simulink model "testing_gyro"  (R2016b)
settings: Solver=FixedStepAuto  StartTime=0.0  StopTime=inf  RelTol=1e-3  EnableMultiTasking=on
libraries: legoev3lib x3
settings Model: SimulationMode=external  ExtModeTrigDuration=2  Creator=Shobhit  LastModifiedBy=karanverma
settings SolverCC: PositivePriorityOrder=on
settings OptimizationCC: LifeSpan=1  MaxStackSize=64
settings DebuggingCC: SFUnexpectedBacktrackingDiag=warning  SFNoUnconditionalDefaultTransitionDiag=warning  SFExecutionAtInitializationDiag=none
settings HardwareCC: ProdBitPerPointer=32  ProdBitPerSizeT=32  ProdBitPerPtrDiffT=32  ProdLargestAtomicInteger=Long  ProdWordSize=32  ProdHWDeviceType=ARM Compatible->ARM 9  UseEmbeddedCoderFeatures=off  UseSimulinkCoderFeatures=off
settings RTWCC: SystemTargetFile=ert.tlc  HardwareBoard=LEGO MINDSTORMS EV3  TLCOptions=-aInlineSetEventsForThisBaseRateFcn=TLC_FALSE -aSuppressMultiTaskScheduler=TLC_FALSE -aRateBasedStepFcn=0  TemplateMakefile=ert_default_tmf  Description=Embedded Coder  GenerateReport=on  Toolchain=Sourcery G++ Lite v2009q3  LaunchReport=on
settings CodeAppCC: ForceParamTrailComments=on  OperatorAnnotations=on  MangleLength=10  MATLABSourceComments=on
settings ERTTargetCC: ERTCustomFileBanners=off  SupportContinuousTime=on  SupportNonInlinedSFcns=on  RemoveResetFunc=off  SupportVariableSizeSignals=on  ModelStepFunctionPrototypeControlCompliant=off
settings ConfigComp: CovMetricSettings=dw  CovHtmlReporting=on  CovSaveCumulativeToWorkspaceVar=on  CovSaveSingleToWorkspaceVar=on  CovExternalEMLEnable=off

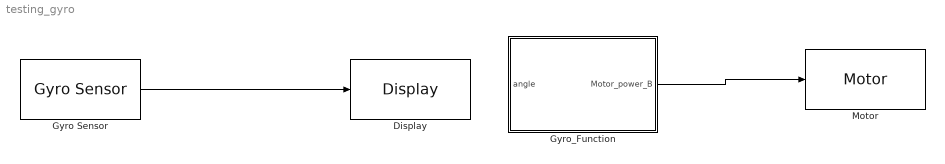
== system testing_gyro ==
  Display : legoev3lib/Display  slcdLine=1  slcdFormat=Decimal
  Gyro Sensor : legoev3lib/Gyro Sensor  portNumber=1  sampleTime=0.1
  Gyro_Function : MATLAB Function  TreatAsAtomicUnit=on
  Motor : legoev3lib/Motor  sportNumber=B  sstopAction=Brake
  wires:
  Gyro Sensor/1 -> Display/1
  Gyro_Function/1(Motor_power_B) -> Motor/1

== matlab function testing_gyro/Gyro_Function ==
  data: angle input; Motor_power_B output
function Motor_power_B = fcn(angle)
if (angle<0)
    Motor_power_B = 20;

else    
     Motor_power_B = 0;
end
